simulink model "line_follower"  (R2018a)
settings: Solver=FixedStepAuto  StartTime=0.0  StopTime=inf  RelTol=1e-3  EnableMultiTasking=on
libraries: arduinolib x12, simulink x1
settings Model: ExtModeTrigDuration=2  Creator=Kushal  LastModifiedBy=RUPAM
settings OptimizationCC: EnhancedBackFolding=on  PassReuseOutputArgsThreshold=0  MaxStackSize=64  OptimizeBlockOrder=speed  DifferentSizesBufferReuse=on  OptimizationCustomize=off
settings DebuggingCC: ParameterTunabilityLossMsg=error
settings HardwareCC: ProdBitPerInt=16  ProdBitPerPointer=16  ProdBitPerSizeT=16  ProdBitPerPtrDiffT=16  ProdLargestAtomicFloat=None  ProdWordSize=8  ProdHWDeviceType=Atmel->AVR  UseEmbeddedCoderFeatures=off
settings SFSimCC: MATLABDynamicMemAlloc=off
settings RTWCC: SystemTargetFile=ert.tlc  HardwareBoard=Arduino Uno  TLCOptions=-aInlineSetEventsForThisBaseRateFcn=TLC_FALSE -aSuppressMultiTaskScheduler=TLC_FALSE -aRateBasedStepFcn=1  TemplateMakefile=ert_default_tmf  GenerateReport=on  Toolchain=Arduino AVR  BuildConfiguration=Faster Runs  LaunchReport=on
settings CodeAppCC: ForceParamTrailComments=on  OperatorAnnotations=on
settings ERTTargetCC: ERTCustomFileBanners=off  SupportContinuousTime=on  SupportNonInlinedSFcns=on  RemoveResetFunc=off  SupportVariableSizeSignals=on  ModelStepFunctionPrototypeControlCompliant=off  ExtMode=on  ExtModeMexArgs='127.0.0.1' 0 17725  ERTSrcFileBannerTemplate=codertarget_code_template.cgt  ERTHdrFileBannerTemplate=codertarget_code_template.cgt  ERTDataSrcFileTemplate=codertarget_code_template.cgt  ERTDataHdrFileTemplate=codertarget_code_template.cgt

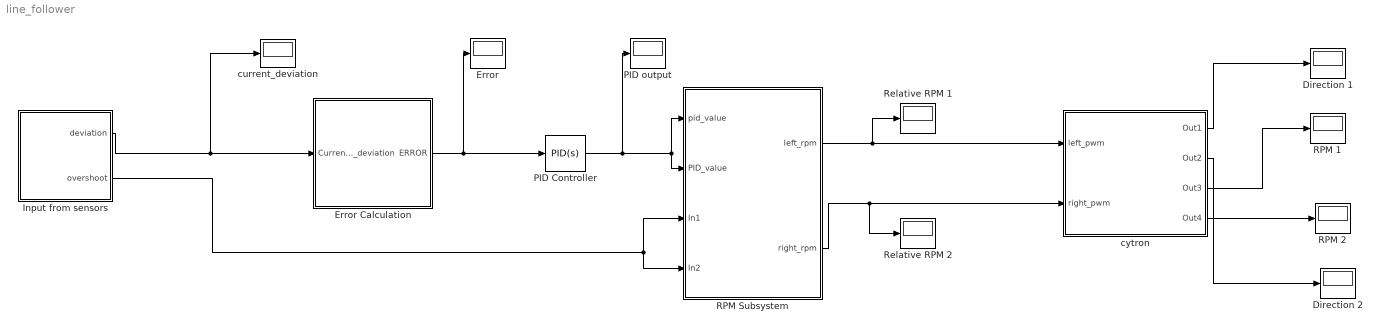
== system line_follower ==
  Direction 1 : Display
  Direction 2 : Display
  Error : Display
  Error Calculation : Subsystem
  "Input from sensors " : Subsystem
  PID Controller : simulink/Continuous/PID Controller  Controller=PID  TimeDomain=Continuous-time  SampleTime=-1  IntegratorMethod=Forward Euler  FilterMethod=Forward Euler  Form=Parallel  UseFilter=on  ControllerParametersSource=internal  P=35  I=0  D=5  N=0  InitialConditionSource=internal  InitialConditionForIntegrator=0  InitialConditionForFilter=0  ExternalReset=none  LimitOutput=off  UpperSaturationLimit=inf  LowerSaturationLimit=-inf  LinearizeAsGain=on  AntiWindupMode=none  Kb=1  TrackingMode=off  Kt=1  PParamMin=[]  PParamMax=[]  IParamMin=[]  IParamMax=[]  DParamMin=[]  DParamMax=[]  NParamMin=[]  NParamMax=[]  KbParamMin=[]  KbParamMax=[]  KtParamMin=[]  KtParamMax=[]  POutMin=[]  POutMax=[]  IOutMin=[]  IOutMax=[]  DOutMin=[]  DOutMax=[]  NOutMin=[]  NOutMax=[]  KbOutMin=[]  KbOutMax=[]  KtOutMin=[]  KtOutMax=[]  IntegratorOutMin=[]  IntegratorOutMax=[]  FilterOutMin=[]  FilterOutMax=[]  SumOutMin=[]  SumOutMax=[]  SumI1OutMin=[]  SumI1OutMax=[]  SumI2OutMin=[]  SumI2OutMax=[]  SumI3OutMin=[]  SumI3OutMax=[]  SumDOutMin=[]  SumDOutMax=[]  SaturationOutMin=[]  SaturationOutMax=[]  IntegratorContinuousStateAttributes=''  IntegratorStateMustResolveToSignalObject=off  IntegratorRTWStateStorageClass=Auto  FilterContinuousStateAttributes=''  FilterStateMustResolveToSignalObject=off  FilterRTWStateStorageClass=Auto  DifferentiatorICPrevScaledInput=0  DifferentiatorOutMin=[]  DifferentiatorOutMax=[]  FilterDiffOutCoefMin=[]  FilterDiffOutCoefMax=[]  SumDenOutMin=[]  SumDenOutMax=[]  SumNumOutMin=[]  SumNumOutMax=[]  ReciprocalOutMin=[]  ReciprocalOutMax=[]  DivideOutMin=[]  DivideOutMax=[]  TunerSelectOption=Transfer Function Based (PID Tuner App)
  PID output : Display
  RPM 1 : Display
  RPM 2 : Display
  RPM Subsystem : Subsystem
  Relative RPM 1 : Display
  Relative RPM 2 : Display
  current_deviation : Display
  cytron : Subsystem
  wires:
  RPM Subsystem/1(left_rpm) -> cytron/1(left_pwm), Relative RPM 1/1
  cytron/1(Out1) -> Direction 1/1
  RPM Subsystem/2(right_rpm) -> Relative RPM 2/1, cytron/2(right_pwm)
  cytron/2(Out2) -> Direction 2/1
  cytron/3(Out3) -> RPM 1/1
  "Input from sensors "/2("overshoot ") -> RPM Subsystem/4(In2), RPM Subsystem/3(In1)
  cytron/4(Out4) -> RPM 2/1
  Error Calculation/1(ERROR) -> Error/1, PID Controller/1
  "Input from sensors "/1(deviation) -> Error Calculation/1(Current_deviation), current_deviation/1
  PID Controller/1 -> PID output/1, RPM Subsystem/1(pid_value), RPM Subsystem/2(PID_value)

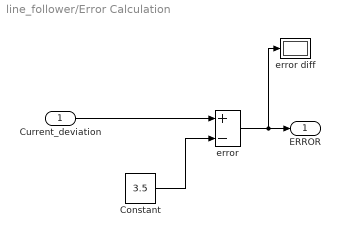
== system line_follower/Error Calculation ==
  Current_deviation : Inport
  Constant : Constant  Value=3.5
  "error " : Sum  Inputs=+-
  error diff : Display
  ERROR : Outport
  wires:
  Current_deviation/1 -> "error "/1
  "error "/1 -> ERROR/1, error diff/1
  Constant/1 -> "error "/2

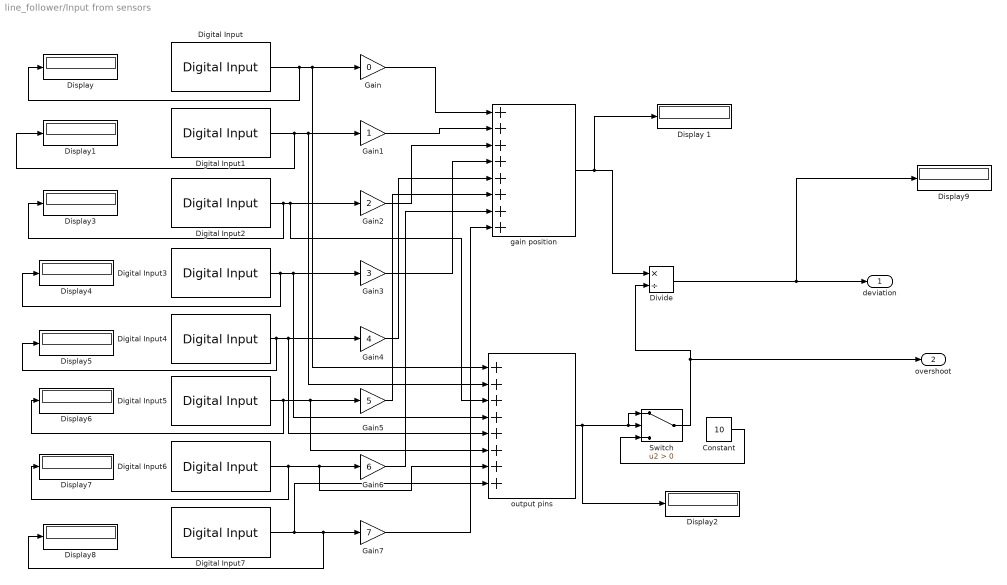
== system line_follower/Input from sensors  ==
  Constant : Constant  Value=10
  Digital Input : arduinolib/Digital Input  pinNumber=2  sampleTime=0.1  blockPlatform=arduino
      settings: SourceProductName=Simulink Support Package for Arduino Hardware
  Digital Input1 : arduinolib/Digital Input  pinNumber=3  sampleTime=0.1  blockPlatform=arduino
      settings: SourceProductName=Simulink Support Package for Arduino Hardware
  Digital Input2 : arduinolib/Digital Input  pinNumber=4  sampleTime=0.1  blockPlatform=arduino
      settings: SourceProductName=Simulink Support Package for Arduino Hardware
  Digital Input3 : arduinolib/Digital Input  pinNumber=7  sampleTime=0.1  blockPlatform=arduino
      settings: SourceProductName=Simulink Support Package for Arduino Hardware
  Digital Input4 : arduinolib/Digital Input  pinNumber=8  sampleTime=0.1  blockPlatform=arduino
      settings: SourceProductName=Simulink Support Package for Arduino Hardware
  Digital Input5 : arduinolib/Digital Input  pinNumber=9  sampleTime=0.1  blockPlatform=arduino
      settings: SourceProductName=Simulink Support Package for Arduino Hardware
  Digital Input6 : arduinolib/Digital Input  pinNumber=10  sampleTime=0.1  blockPlatform=arduino
      settings: SourceProductName=Simulink Support Package for Arduino Hardware
  Digital Input7 : arduinolib/Digital Input  pinNumber=11  sampleTime=0.1  blockPlatform=arduino
      settings: SourceProductName=Simulink Support Package for Arduino Hardware
  Display{,1..9} (10 alike) : Display
  Display 1 : Display
  Divide : Product  Inputs=*/
  Gain : Gain  Gain=0
  Gain1 : Gain
  Gain2 : Gain  Gain=2
  Gain3 : Gain  Gain=3
  Gain4 : Gain  Gain=4
  Gain5 : Gain  Gain=5
  Gain6 : Gain  Gain=6
  Gain7 : Gain  Gain=7
  Switch : Switch  Criteria=u2 > Threshold
  gain position : Sum  Inputs=++++++++  OutMax=[30]
  output pins : Sum  Inputs=++++++++  OutMax=[9]
  deviation : Outport
  "overshoot " : Outport  Port=2
  wires:
  Digital Input6/1 -> Display7/1, output pins/7, Gain6/1
  Digital Input1/1 -> Display1/1, output pins/2, Gain1/1
  Gain1/1 -> gain position/2
  Gain4/1 -> gain position/5
  Digital Input2/1 -> Display3/1, output pins/3, Gain2/1
  Digital Input7/1 -> output pins/8, Display8/1, Gain7/1
  Gain/1 -> gain position/1
  Gain2/1 -> gain position/3
  Digital Input5/1 -> Display6/1, output pins/6, Gain5/1
  Digital Input4/1 -> output pins/5, Gain4/1, Display5/1
  Gain7/1 -> gain position/8
  Gain5/1 -> gain position/6
  Gain3/1 -> gain position/4
  Digital Input/1 -> Display/1, output pins/1, Gain/1
  gain position/1 -> Display 1/1, Divide/1
  Digital Input3/1 -> output pins/4, Gain3/1, Display4/1
  Gain6/1 -> gain position/7
  output pins/1 -> Display2/1, Switch/1, Switch/2
  Switch/1 -> Divide/2, "overshoot "/1
  Constant/1 -> Switch/3
  Divide/1 -> Display9/1, deviation/1

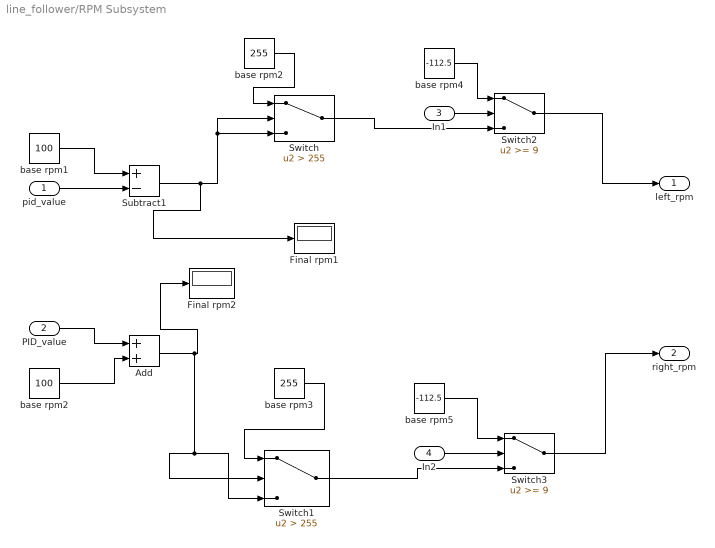
== system line_follower/RPM Subsystem ==
  pid_value : Inport
  PID_value : Inport  Port=2
  In1 : Inport  Port=3
  In2 : Inport  Port=4
  Add : Sum
  Final rpm1 : Display
  "Final rpm2 " : Display
  Subtract1 : Sum  Inputs=+-
  Switch : Switch  Criteria=u2 > Threshold  Threshold=255
  Switch1 : Switch  Criteria=u2 > Threshold  Threshold=255
  Switch2 : Switch  Threshold=9
  Switch3 : Switch  Threshold=9
  base rpm1 : Constant  Value=100
  base rpm2 : Constant  Value=255
  "base rpm2 " : Constant  Value=100
  base rpm3 : Constant  Value=255
  base rpm4 : Constant  Value=-112.5
  base rpm5 : Constant  Value=-112.5
  left_rpm : Outport
  right_rpm : Outport  Port=2
  wires:
  pid_value/1 -> Subtract1/2
  "base rpm2 "/1 -> Add/2
  Subtract1/1 -> Switch/3, Switch/2, Final rpm1/1
  base rpm1/1 -> Subtract1/1
  PID_value/1 -> Add/1
  Add/1 -> "Final rpm2 "/1, Switch1/2, Switch1/3
  base rpm2/1 -> Switch/1
  base rpm3/1 -> Switch1/1
  In1/1 -> Switch2/2
  In2/1 -> Switch3/2
  Switch2/1 -> left_rpm/1
  Switch3/1 -> right_rpm/1
  Switch1/1 -> Switch3/3
  Switch/1 -> Switch2/3
  base rpm4/1 -> Switch2/1
  base rpm5/1 -> Switch3/1

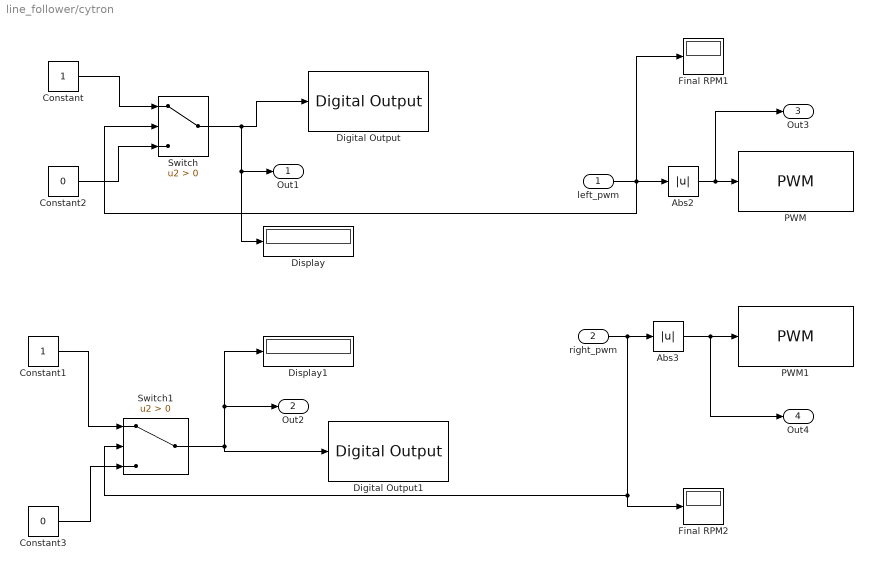
== system line_follower/cytron ==
  left_pwm : Inport
  right_pwm : Inport  Port=2
  Abs2 : Abs
  Abs3 : Abs
  Constant : Constant
  Constant1 : Constant
  Constant2 : Constant  Value=0
  Constant3 : Constant  Value=0
  Digital Output : arduinolib/Digital Output  pinNumber=13  blockPlatform=arduino
  Digital Output1 : arduinolib/Digital Output  pinNumber=12  blockPlatform=arduino
  Display : Display
  Display1 : Display
  "Final RPM1 " : Display
  "Final RPM2 " : Display
  PWM : arduinolib/PWM  pinNumber=5  EnableInputFrequency=off  InitialFrequency=2000  InitialDutyCycle=0  NotificationType=None  blockPlatform=arduino
  PWM1 : arduinolib/PWM  pinNumber=6  EnableInputFrequency=off  InitialFrequency=2000  InitialDutyCycle=0  NotificationType=None  blockPlatform=arduino
  Switch : Switch  Criteria=u2 > Threshold
  Switch1 : Switch  Criteria=u2 > Threshold
  Out1 : Outport
  Out2 : Outport  Port=2
  Out3 : Outport  Port=3
  Out4 : Outport  Port=4
  wires:
  Constant/1 -> Switch/1
  Switch/1 -> Out1/1, Display/1, Digital Output/1
  Constant1/1 -> Switch1/1
  Abs2/1 -> Out3/1, PWM/1
  Abs3/1 -> Out4/1, PWM1/1
  Switch1/1 -> Out2/1, Display1/1, Digital Output1/1
  Constant2/1 -> Switch/3
  Constant3/1 -> Switch1/3
  left_pwm/1 -> "Final RPM1 "/1, Switch/2, Abs2/1
  right_pwm/1 -> "Final RPM2 "/1, Switch1/2, Abs3/1
